simulink model "ESO_1"  (Simulink 7.9)
settings: Solver=ode45  StartTime=0.0  StopTime=10.0  RelTol=1e-3
values from neighbouring files (symbols this model uses):
  K01 = diag([6,6,6])    [constant.m]
  K02 = diag([8,8,8])    [constant.m]
  K03 = diag([16,16,16])    [constant.m]
  M = diag([m11,m22,m33])    [constant.m]    (also in ship_plant.m)
settings Model: Creator=Administrator  LastModifiedBy=Administrator

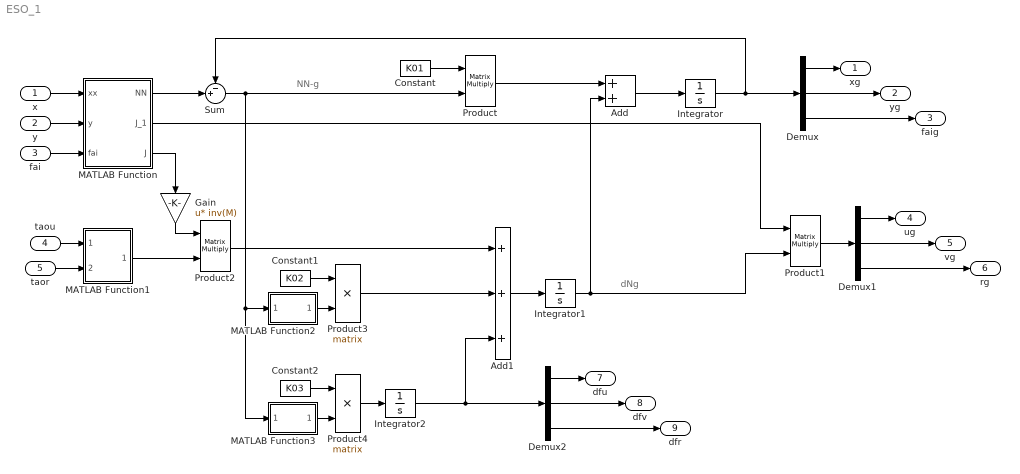
== system ESO_1 ==
  note: NN-g
  note: dNg
  x : Inport
  y : Inport  Port=2
  fai : Inport  Port=3
  taou : Inport  Port=4
  taor : Inport  Port=5
  Add : Sum
  Add1 : Sum  Inputs=+++
  Constant : Constant  Value=K01
  Constant1 : Constant  Value=K02
  Constant2 : Constant  Value=K03
  Demux : Demux  Outputs=3
  Demux1 : Demux  Outputs=3
  Demux2 : Demux  Outputs=3
  Gain : Gain  Gain=inv(M)  Multiplication=Matrix(u*K)
  Integrator : Integrator
  Integrator1 : Integrator
  Integrator2 : Integrator
  MATLAB Function : MATLAB Function  TreatAsAtomicUnit=on
  MATLAB Function1 : MATLAB Function  TreatAsAtomicUnit=on
  MATLAB Function2 : MATLAB Function  TreatAsAtomicUnit=on
  MATLAB Function3 : MATLAB Function  TreatAsAtomicUnit=on
  Product{,1..4} (5 alike) : Product  Multiplication=Matrix(*)  RndMeth=Zero
  Sum : Sum  Inputs=-+|
  xg : Outport
  yg : Outport  Port=2
  faig : Outport  Port=3
  ug : Outport  Port=4
  vg : Outport  Port=5
  rg : Outport  Port=6
  dfu : Outport  Port=7
  dfv : Outport  Port=8
  dfr : Outport  Port=9
  wires:
  x/1 -> MATLAB Function/1(xx)
  y/1 -> MATLAB Function/2(y)
  fai/1 -> MATLAB Function/3(fai)
  Sum/1 -> Product/2, MATLAB Function2/1(ETA), MATLAB Function3/1(ETA)
  MATLAB Function/1(NN) -> Sum/2
  Integrator/1 -> Sum/1, Demux/1
  Constant/1 -> Product/1
  Product/1 -> Add/1
  Integrator1/1 -> Product1/2, Add/2
  Add/1 -> Integrator/1
  Demux/1 -> xg/1
  Demux/2 -> yg/1
  Demux/3 -> faig/1
  MATLAB Function/3(J) -> Gain/1
  MATLAB Function/2(J_1) -> Product1/1
  Add1/1 -> Integrator1/1
  taou/1 -> MATLAB Function1/1(taou)
  taor/1 -> MATLAB Function1/2(taor)
  MATLAB Function1/1(TAO) -> Product2/2
  Gain/1 -> Product2/1
  Product2/1 -> Add1/1
  Constant1/1 -> Product3/1
  MATLAB Function2/1(FAL) -> Product3/2
  Product3/1 -> Add1/2
  Constant2/1 -> Product4/1
  MATLAB Function3/1(FAL) -> Product4/2
  Product4/1 -> Integrator2/1
  Integrator2/1 -> Add1/3, Demux2/1
  Demux1/1 -> ug/1
  Demux1/2 -> vg/1
  Demux1/3 -> rg/1
  Product1/1 -> Demux1/1
  Demux2/1 -> dfu/1
  Demux2/2 -> dfv/1
  Demux2/3 -> dfr/1

== matlab function MATLAB Function1 ==
  data: taou input double; TAO output double; taor input double
function TAO = fcn(taou,taor)
%#codegen
TAO=[taou;0;taor];

== matlab function MATLAB Function ==
  data: xx input double; y input double; fai input double; NN output double; J_1 output double; J output double
function [NN,J_1,J]= fcn(xx,y,fai)
%#codegen
NN=[xx;y;fai];
J=[cos(fai) -sin(fai) 0;
    sin(fai) cos(fai) 0;
    0 0 1];
J_1=inv(J);

== matlab function MATLAB Function2 ==
  data: ETA input double; FAL output double
function FAL = fcn(ETA)
%#codegen
x1=[1 0 0]*ETA;
x2=[0 1 0]*ETA;
x3=[0 0 1]*ETA;
% y1=(abs(x1))^(1/2)*sign(x1);
% y2=(abs(x2))^(1/2)*sign(x2);
% y3=(abs(x3))^(1/2)*sign(x3);
% YY2 = [y1;y2;y3];
a1=0.5;deta1=0.001;
if abs(x1)>deta1
    fal1=abs(x1)^a1*sign(x1);
else
    fal1=x1/(deta1^(1-a1));
end
a2=0.5;deta2=0.001;
if abs(x2)>deta1
    fal2=abs(x2)^a2*sign(x2);
else
    fal2=x2/(deta2^(1-a2));
end
a3=0.5;deta3=0.01;
if abs(x3)>deta3
    fal3=abs(x3)^a3*sign(x3);
else
    fal3=x3/(deta3^(1-a3));
end
FAL=[fal1;fal2;fal3];

== matlab function MATLAB Function3 ==
  data: ETA input double; FAL output double
function FAL = fcn(ETA)
%#codegen
x1=[1 0 0]*ETA;
x2=[0 1 0]*ETA;
x3=[0 0 1]*ETA;
% y1=(abs(x1))^(1/2)*sign(x1);
% y2=(abs(x2))^(1/2)*sign(x2);
% y3=(abs(x3))^(1/2)*sign(x3);
% YY2 = [y1;y2;y3];
a1=0.5;deta1=0.001;
if abs(x1)>deta1
    fal1=abs(x1)^a1*sign(x1);
else
    fal1=x1/(deta1^(1-a1));
end
a2=0.5;deta2=0.001;
if abs(x2)>deta1
    fal2=abs(x2)^a2*sign(x2);
else
    fal2=x2/(deta2^(1-a2));
end
a3=0.5;deta3=0.01;
if abs(x3)>deta3
    fal3=abs(x3)^a3*sign(x3);
else
    fal3=x3/(deta3^(1-a3));
end
FAL=[fal1;fal2;fal3];
